simulink model "comb"  (R2023a)
settings: Solver=VariableStepAuto  StartTime=0.0  StopTime=10.0  RelTol=1e-3
undefined symbols (not defined in the file): m
libraries: dspsrcs4 x1, dspxfrm3 x1
settings Model: Creator=ricca  LastModifiedBy=ricca

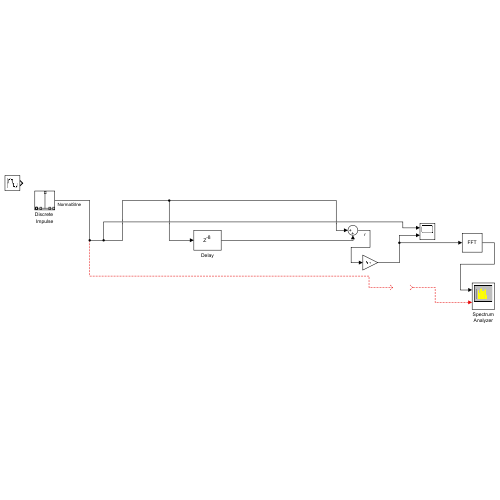
[thumbnail: Simulink's stored preview of the top-level diagram]
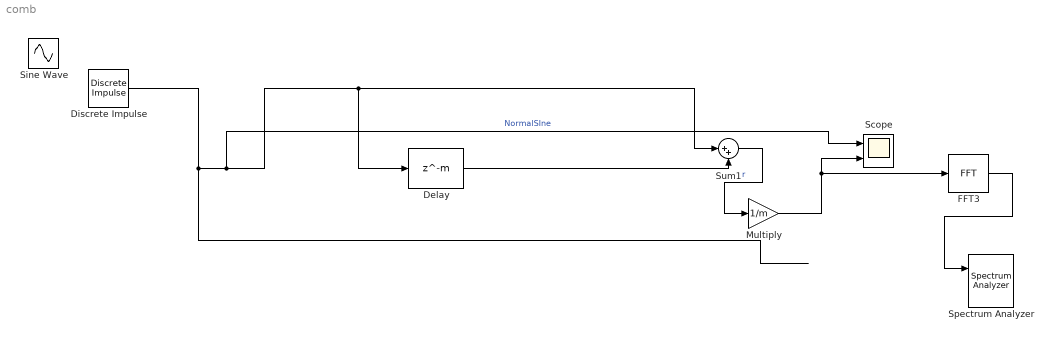
== system comb ==
  Delay : Delay  DelayLength=m  InitialCondition=0  UseCircularBuffer=on
  Discrete Impulse : dspsrcs4/Discrete  Impulse  Delay=0  SampleTime=0.001  FrameSample=1  OutputFrames=off  dataType=double  isSigned=on  wordLen=16  udDataType=sfix(16)  fracBitsMode=Best precision  numFracBits=15  OutDataTypeStr=double  LastOutDataTypeStr=double
  FFT3 : dspxfrm3/FFT  FFTImplementation=Auto  CompMethod=Table lookup  TableOpt=NEW  TableOptActive=Speed  BitRevOrder=off  Normalize=off  InheritFFTLength=on  FFTLength=64  WrapInput=on  roundingMode=Floor  overflowMode=off  firstCoeffDataTypeStr=Inherit: Same word length as input  firstCoeffLastDataTypeStr=Inherit: Same word length as input  outputMin=[]  outputMax=[]
  Multiply : Gain  Gain=1/m
  Scope : Scope  NumInputPorts=2
  Sine Wave : Sin  Frequency=1000  SampleTime=0.001
  Spectrum Analyzer : SpectrumAnalyzer  NumInputPorts=2  WindowPosition=[368.000000,182.000000,800.000000,500.000000,]  ScopeFrameLocation=window  Span=1000  StartFrequency=-500  StopFrequency=500  YLimits=[-104.84025466,-31.67638683]  ColorLimits=[-104.84025466,-31.67638683]  ShowLegend=on  DefaultConfigurationName=spbscopes.SpectrumAnalyzerBlockCfg  IsFrequencyInputMode=0  FrequencyVectorPort=0  FrequencyVectorFromPort=0  FrequencyInputRBWPort=0  FrequencyInputRBWFromPort=0
  Sum1 : Sum  Inputs=|++
  wires:
  Discrete Impulse/1 -> Sum1/1, Delay/1, Scope/1  "NormalSIne"
  Delay/1 -> Sum1/2
  Sum1/1 -> Multiply/1  "r"
  ? -> Spectrum Analyzer/2
  FFT3/1 -> Spectrum Analyzer/1
  Multiply/1 -> FFT3/1, Scope/2
